simulink model "simulator"  (R2024a)
settings: Solver=VariableStepAuto  StartTime=0.0  StopTime=10  RelTol=1e-3
values from neighbouring files (symbols this model uses):
  params = struct()    [Data.m]
libraries: simulink x2, matrix_library x1
settings Model: Creator=matteocolussi  LastModifiedBy=matteocolussi

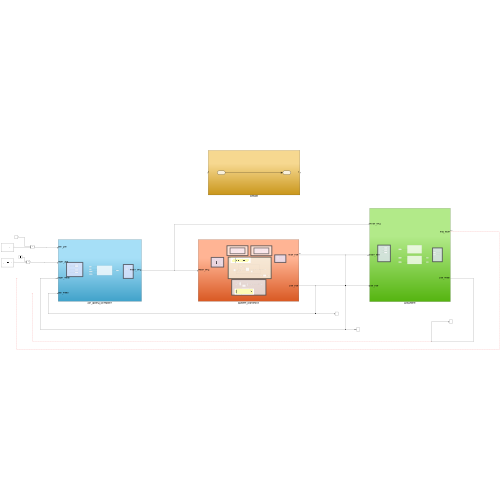
[thumbnail: Simulink's stored preview of the top-level diagram]
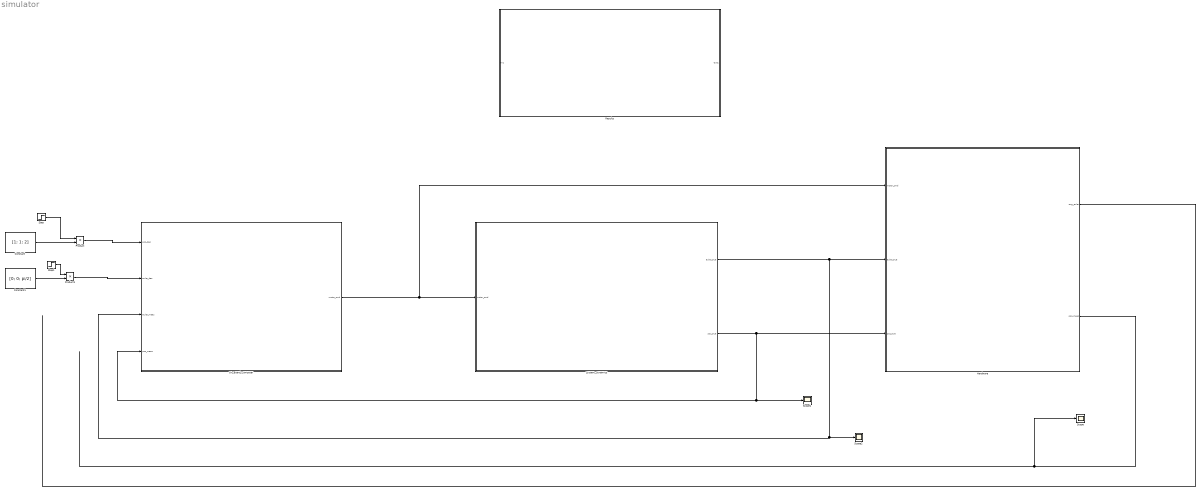
== system simulator ==
  Constant : Constant  Value=[1; 1; 2]
  Constant1 : Constant  Value=[0; 0; pi/2]
  Hardware : Subsystem
  On_Board_Computer : Subsystem
  Product : Product
  Product1 : Product
  Results : Subsystem
  Scope : Scope
  Scope1 : Scope
  Scope2 : Scope
  Step : Step  Time=0  SampleTime=0
  Step1 : Step  Time=0  SampleTime=0
  System_Dynamics : Subsystem
  wires:
  On_Board_Computer/1(motor_cmd) -> Hardware/1(motor_cmd), System_Dynamics/1(motor_cmd)
  System_Dynamics/1(euler_true) -> Hardware/2(euler_true), On_Board_Computer/3(euler_meas), Scope2/1
  System_Dynamics/2(pos_true) -> Scope1/1, On_Board_Computer/4(pos_meas), Hardware/3(pos_true)
  Hardware/1(ang_euler) -> ?
  Hardware/2(pos_meas) -> Scope/1
  Constant/1 -> Product/2
  Step/1 -> Product/1
  Product/1 -> On_Board_Computer/1(pos_des)
  Constant1/1 -> Product1/2
  Step1/1 -> Product1/1
  Product1/1 -> On_Board_Computer/2(euler_des)

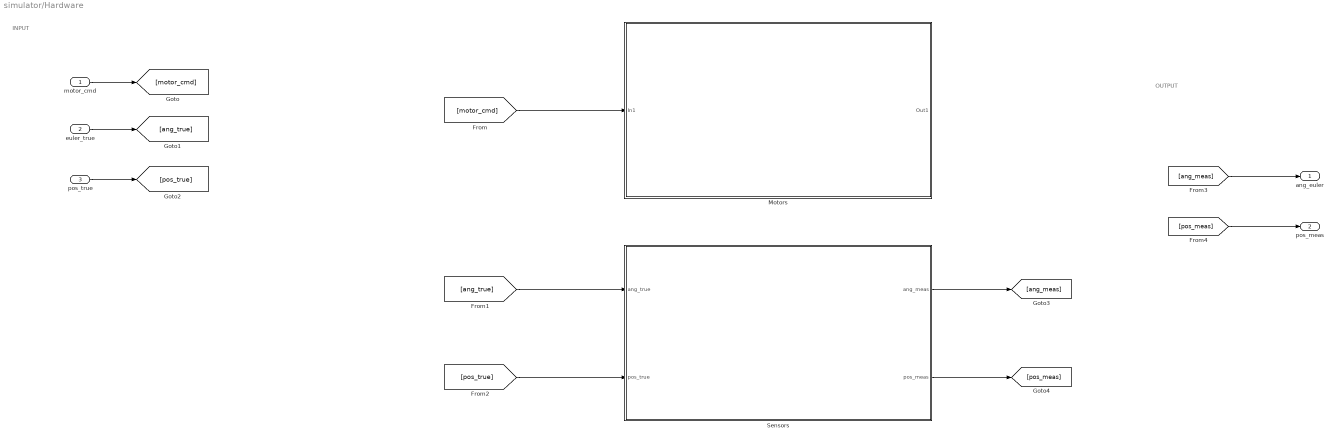
== system simulator/Hardware ==
  note: INPUT
  note: OUTPUT
  motor_cmd : Inport
  euler_true : Inport  Port=2
  pos_true : Inport  Port=3
  Motors : Subsystem
  Sensors : Subsystem
  ang_euler : Outport
  pos_meas : Outport  Port=2
  wires:
  motor_cmd/1 -> [motor_cmd]
  [motor_cmd] -> Motors/1(In1)
  euler_true/1 -> [ang_true]
  pos_true/1 -> [pos_true]
  [ang_true] -> Sensors/1(ang_true)
  [pos_true] -> Sensors/2(pos_true)
  Sensors/1(ang_meas) -> [ang_meas]
  Sensors/2(pos_meas) -> [pos_meas]
  [ang_meas] -> ang_euler/1
  [pos_meas] -> pos_meas/1

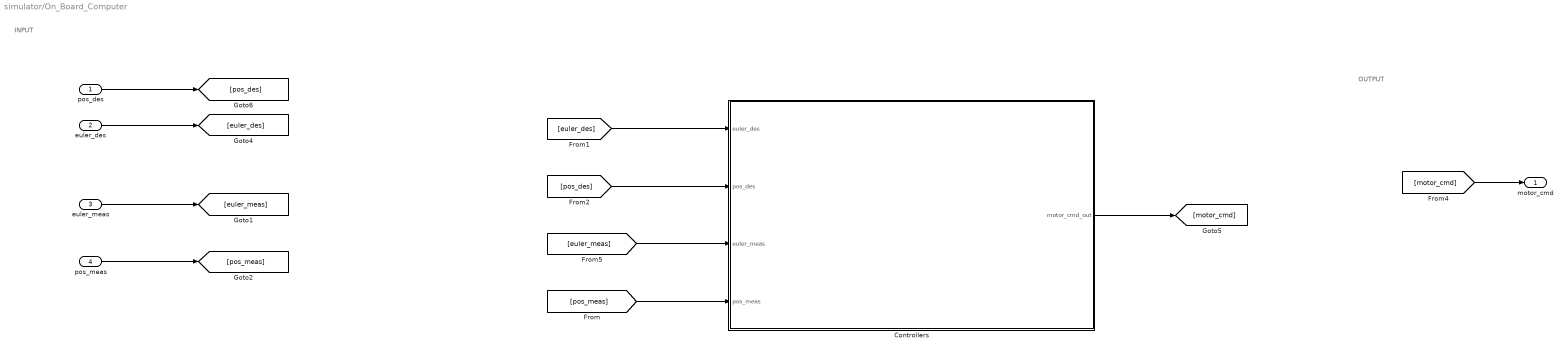
== system simulator/On_Board_Computer ==
  note: OUTPUT
  note: INPUT
  pos_des : Inport
  euler_des : Inport  Port=2
  euler_meas : Inport  Port=3
  pos_meas : Inport  Port=4
  Controllers : Subsystem
  motor_cmd : Outport
  wires:
  pos_des/1 -> [pos_des]
  [euler_des] -> Controllers/1(euler_des)
  [pos_des] -> Controllers/2(pos_des)
  euler_des/1 -> [euler_des]
  Controllers/1(motor_cmd_out) -> [motor_cmd]
  [motor_cmd] -> motor_cmd/1
  euler_meas/1 -> [euler_meas]
  pos_meas/1 -> [pos_meas]
  [pos_meas] -> Controllers/4(pos_meas)
  [euler_meas] -> Controllers/3(euler_meas)

== system simulator/Results ==
  In1 : Inport
  Out1 : Outport
  wires:
  In1/1 -> Out1/1

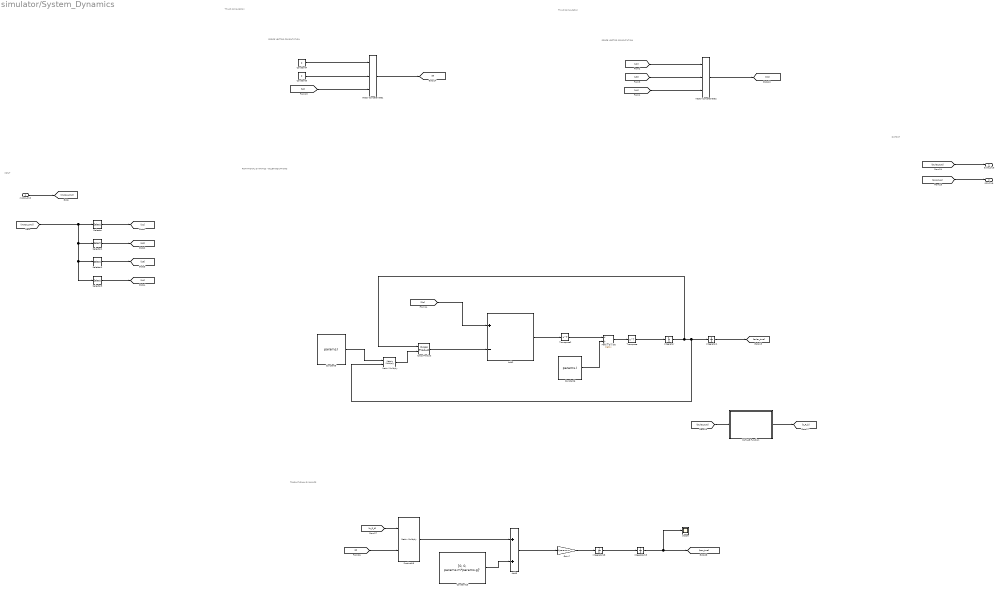
== system simulator/System_Dynamics ==
  note: ROTATIONAL DYNAMICS - EULER EQUATIONS
  note: FORCE VECTOR COMPUTATION
  note: Thrust computation
  note: INPUT
  note: OUTPUT
  note: TRASLATIONAL DYNAMICS
  note: Thrust computation
  note: FORCE VECTOR COMPUTATION
  motor_cmd : Inport
  Add2 : Sum  Inputs=+-
  Add6 : Sum
  Constant13 : Constant  Value=[0, 0, params.m*params.g]'
  Constant3 : Constant  Value=0
  Constant4 : Constant  Value=0
  Constant5 : Constant  Value=params.I  VectorParams1D=off
  Constant6 : Constant  Value=params.I
  Cross Product : matrix_library/Cross Product
  Gain7 : Gain  Gain=1/params.m
  Integrator{,1,18..19} (4 alike) : Integrator
  MATLAB Function : MATLAB Function  TreatAsAtomicUnit=on
  Matrix Divide : Product  Inputs=*/  Multiplication=Matrix(*)
  Matrix Multiply : Product  Multiplication=Matrix(*)
  Product18 : Product  Multiplication=Matrix(*)
  Scope : Scope
  Selector : Selector  InputPortWidth=4  IndexOptions=Index vector (dialog)  Indices=1  OutputSizes=1
  Selector1 : Selector  InputPortWidth=4  IndexOptions=Index vector (dialog)  Indices=2  OutputSizes=1
  Selector2 : Selector  InputPortWidth=4  IndexOptions=Index vector (dialog)  Indices=3  OutputSizes=1
  Selector3 : Selector  InputPortWidth=4  IndexOptions=Index vector (dialog)  Indices=4  OutputSizes=1
  Transpose : Math  Operator=transpose
  Transpose2 : Math  Operator=transpose
  Vector Concatenate1 : Concatenate  NumInputs=3
  Vector Concatenate2 : Concatenate  NumInputs=3
  euler_true : Outport
  pos_true : Outport  Port=2
  wires:
  motor_cmd/1 -> [motor_cmd]
  Selector/1 -> [U1]
  Selector1/1 -> [U2]
  Selector2/1 -> [U3]
  [motor_cmd] -> Selector3/1, Selector2/1, Selector1/1, Selector/1
  Selector3/1 -> [U4]
  [U1] -> Vector Concatenate1/3
  Constant3/1 -> Vector Concatenate1/2
  Constant4/1 -> Vector Concatenate1/1
  Vector Concatenate1/1 -> [F]  "Force"
  [euler_true] -> MATLAB Function/1(ang)
  MATLAB Function/1(o_R_b) -> [o_R_b]
  [euler_true] -> euler_true/1
  [pos_true] -> pos_true/1
  Add6/1 -> Gain7/1
  [F] -> Product18/2
  Product18/1 -> Add6/1
  Gain7/1 -> Integrator18/1  "r_dotdot"
  [o_R_b] -> Product18/1
  Constant13/1 -> Add6/2
  Integrator18/1 -> Integrator19/1  "r_dot"
  Integrator19/1 -> [pos_true], Scope/1  "r"
  Constant5/1 -> Matrix Multiply/1
  Matrix Multiply/1 -> Cross Product/2
  Cross Product/1 -> Add2/2
  Add2/1 -> Transpose2/1
  Constant6/1 -> Matrix Divide/2
  Matrix Divide/1 -> Transpose/1  "w_dot"
  Integrator/1 -> Cross Product/1, Matrix Multiply/2, Integrator1/1  "w"
  Integrator1/1 -> [euler_true]  "euler_angles"
  [U2] -> Vector Concatenate2/1
  Vector Concatenate2/1 -> [Mc]  "Torque"
  [U4] -> Vector Concatenate2/3
  [U3] -> Vector Concatenate2/2
  Transpose/1 -> Integrator/1
  [Mc] -> Add2/1
  Transpose2/1 -> Matrix Divide/1

== system simulator/Hardware/Motors ==
  In1 : Inport
  Out1 : Outport
  wires:
  In1/1 -> Out1/1

== system simulator/Hardware/Sensors ==
  note: OUTPUT
  note: INPUT
  ang_true : Inport
  pos_true : Inport  Port=2
  MPU6050 : Subsystem
  ang_meas : Outport
  pos_meas : Outport  Port=2
  wires:
  ang_true/1 -> [ang_true]
  pos_true/1 -> [pos_true]
  [ang_meas] -> ang_meas/1
  [pos_meas] -> pos_meas/1
  [ang_true] -> MPU6050/1(ang_true)
  [pos_true] -> MPU6050/2(pos_true)
  MPU6050/1(ang_meas) -> [ang_meas]
  MPU6050/2(pos_meas) -> [pos_meas]

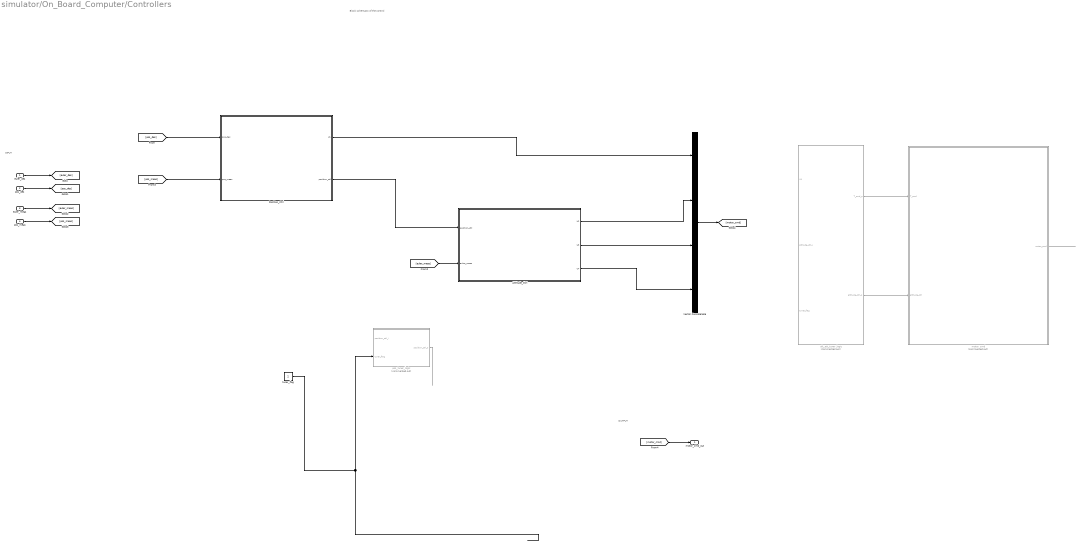
== system simulator/On_Board_Computer/Controllers ==
  note: Block schematic of the control
  note: OUTPUT
  note: INPUT
  euler_des : Inport
  pos_des : Inport  Port=2
  euler_meas : Inport  Port=3
  pos_meas : Inport  Port=4
  Attitude_Ctrl : Subsystem
  Position_Ctrl : Subsystem
  Vector Concatenate : Concatenate  NumInputs=4
  alt_att_tuner_logic : Subsystem  Commented=on
  motor_cmd : Subsystem  Commented=on
  pos_tuner_logic : Subsystem  Commented=on
  tuner_flag : Constant  Value=2
  motor_cmd_out : Outport
  wires:
  euler_des/1 -> [euler_des]
  pos_des/1 -> [pos_des]
  pos_meas/1 -> [pos_meas]
  euler_meas/1 -> [euler_meas]
  [euler_meas] -> Attitude_Ctrl/2(euler_meas)
  motor_cmd/1(motor_cmd) -> ?
  [motor_cmd] -> motor_cmd_out/1
  [pos_meas] -> Position_Ctrl/2(pos_meas)
  tuner_flag/1 -> pos_tuner_logic/2(tuner_flag)
  [pos_des] -> Position_Ctrl/1(pos_des)
  Position_Ctrl/2(position_ctrl) -> Attitude_Ctrl/1(position_ctrl)
  pos_tuner_logic/1(position_ctrl_o) -> ?
  Position_Ctrl/1(U1) -> Vector Concatenate/1
  alt_att_tuner_logic/1(T_cmd_o) -> motor_cmd/1(T_cmd)
  alt_att_tuner_logic/2(attitude_ctrl_o) -> motor_cmd/2(attitude_ctrl)
  Attitude_Ctrl/1(U2) -> Vector Concatenate/2
  Attitude_Ctrl/2(U3) -> Vector Concatenate/3
  Attitude_Ctrl/3(U4) -> Vector Concatenate/4
  Vector Concatenate/1 -> [motor_cmd]

== system simulator/Hardware/Sensors/MPU6050 ==
  note: INPUT
  note: OUTPUT
  ang_true : Inport
  pos_true : Inport  Port=2
  ACCELEROMETER : Subsystem
  GYROSCOPE : Subsystem
  ang_meas : Outport
  pos_meas : Outport  Port=2
  wires:
  ang_true/1 -> [ang_true]
  pos_true/1 -> [pos_true]
  [pos_meas] -> pos_meas/1
  [ang_meas] -> ang_meas/1
  [ang_true] -> GYROSCOPE/1(ang_true)
  [pos_true] -> ACCELEROMETER/1(pos_true)
  GYROSCOPE/1(ang_meas) -> [ang_meas]
  ACCELEROMETER/1(pos_meas) -> [pos_meas]

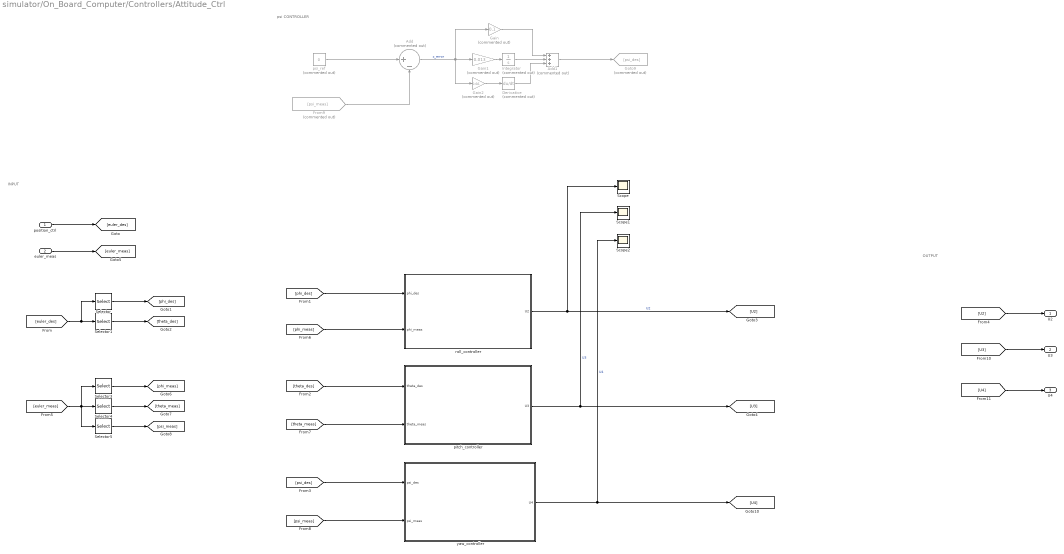
== system simulator/On_Board_Computer/Controllers/Attitude_Ctrl ==
  note: OUTPUT
  note: INPUT
  note: psi CONTROLLER
  position_ctrl : Inport
  euler_meas : Inport  Port=2
  Add : Sum  Commented=on  Inputs=|+-
  Add1 : Sum  Commented=on  Inputs=+++
  Derivative : Derivative  Commented=on
  From9 : From  Commented=on  GotoTag=psi_meas
  Gain : Gain  Commented=on  Gain=0.1
  Gain1 : Gain  Commented=on  Gain=0.013
  Gain2 : Gain  Commented=on  Gain=0.66
  Goto9 : Goto  Commented=on  GotoTag=psi_des
  Integrator : Integrator  Commented=on
  Scope : Scope
  Scope1 : Scope
  Scope2 : Scope
  Selector : Selector  InputPortWidth=2  IndexOptions=Index vector (dialog)  Indices=1  OutputSizes=1
  Selector1 : Selector  InputPortWidth=2  IndexOptions=Index vector (dialog)  Indices=2  OutputSizes=1
  Selector3 : Selector  InputPortWidth=3  IndexOptions=Index vector (dialog)  Indices=1  OutputSizes=1
  Selector4 : Selector  InputPortWidth=3  IndexOptions=Index vector (dialog)  Indices=2  OutputSizes=1
  Selector5 : Selector  InputPortWidth=3  IndexOptions=Index vector (dialog)  Indices=3  OutputSizes=1
  pitch_controller : Subsystem
  psi_ref : Constant  Commented=on  Value=0
  roll_controller : Subsystem
  yaw_controller : Subsystem
  U2 : Outport
  U3 : Outport  Port=2
  U4 : Outport  Port=3
  wires:
  position_ctrl/1 -> [euler_des]
  [phi_des] -> roll_controller/1(phi_des)
  [theta_des] -> pitch_controller/1(theta_des)
  [psi_des] -> yaw_controller/1(psi_des)
  roll_controller/1(U2) -> [U2], Scope/1  "U2"
  pitch_controller/1(U3) -> [U3], Scope1/1  "U3"
  yaw_controller/1(U4) -> [U4], Scope2/1  "U4"
  euler_meas/1 -> [euler_meas]
  [phi_meas] -> roll_controller/2(phi_meas)
  [theta_meas] -> pitch_controller/2(theta_meas)
  [psi_meas] -> yaw_controller/2(psi_meas)
  Selector/1 -> [phi_des]
  [euler_des] -> Selector1/1, Selector/1
  Selector1/1 -> [theta_des]
  [euler_meas] -> Selector5/1, Selector4/1, Selector3/1
  Selector4/1 -> [theta_meas]
  Selector5/1 -> [psi_meas]
  Selector3/1 -> [phi_meas]
  [U2] -> U2/1
  psi_ref/1 -> Add/1
  From9/1 -> Add/2
  [U3] -> U3/1
  [U4] -> U4/1
  Gain1/1 -> Integrator/1
  Integrator/1 -> Add1/2
  Add/1 -> Gain2/1, Gain1/1, Gain/1  "z_error"
  Add1/1 -> Goto9/1
  Gain/1 -> Add1/1
  Derivative/1 -> Add1/3
  Gain2/1 -> Derivative/1

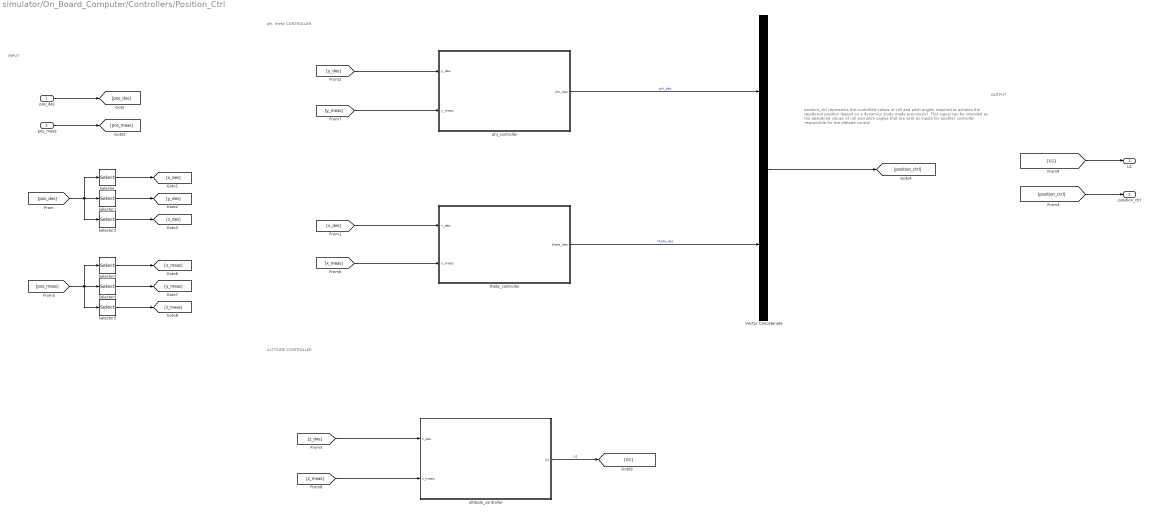
== system simulator/On_Board_Computer/Controllers/Position_Ctrl ==
  note: position_ctrl represents the controlled values of roll and pitch angles required to achieve the desidered position (based on a dynamics study made previously).
      |
      | This signal can be intended as the desidered values of roll and pitch angles that are sent as inputs for another controller, responsible for the attitude control .
  note: ALTITUDE CONTROLLER
  note: phi, theta CONTROLLER
  note: INPUT
  note: OUTPUT
  pos_des : Inport
  pos_meas : Inport  Port=2
  Selector : Selector  InputPortWidth=3  IndexOptions=Index vector (dialog)  Indices=1  OutputSizes=1
  Selector1 : Selector  InputPortWidth=3  IndexOptions=Index vector (dialog)  Indices=2  OutputSizes=1
  Selector2 : Selector  InputPortWidth=3  IndexOptions=Index vector (dialog)  Indices=3  OutputSizes=1
  Selector3 : Selector  InputPortWidth=3  IndexOptions=Index vector (dialog)  Indices=1  OutputSizes=1
  Selector4 : Selector  InputPortWidth=3  IndexOptions=Index vector (dialog)  Indices=2  OutputSizes=1
  Selector5 : Selector  InputPortWidth=3  IndexOptions=Index vector (dialog)  Indices=3  OutputSizes=1
  Vector Concatenate : Concatenate
  altitude_controller : Subsystem
  phi_controller : Subsystem
  theta_controller : Subsystem
  U1 : Outport
  position_ctrl : Outport  Port=2
  wires:
  Selector3/1 -> [x_meas]
  Selector4/1 -> [y_meas]
  [pos_meas] -> Selector5/1, Selector4/1, Selector3/1
  pos_meas/1 -> [pos_meas]
  Selector5/1 -> [z_meas]
  [pos_des] -> Selector2/1, Selector1/1, Selector/1
  Selector/1 -> [x_des]
  pos_des/1 -> [pos_des]
  Selector1/1 -> [y_des]
  Selector2/1 -> [z_des]
  [y_meas] -> phi_controller/2(y_meas)
  [x_des] -> theta_controller/1(x_des)
  [y_des] -> phi_controller/1(y_des)
  [x_meas] -> theta_controller/2(x_meas)
  [position_ctrl] -> position_ctrl/1
  Vector Concatenate/1 -> [position_ctrl]
  theta_controller/1(theta_des) -> Vector Concatenate/2  "theta_des"
  [z_meas] -> altitude_controller/2(z_meas)
  [z_des] -> altitude_controller/1(z_des)
  altitude_controller/1(U1) -> [U1]  "U1"
  [U1] -> U1/1
  phi_controller/1(phi_des) -> Vector Concatenate/1  "phi_des"

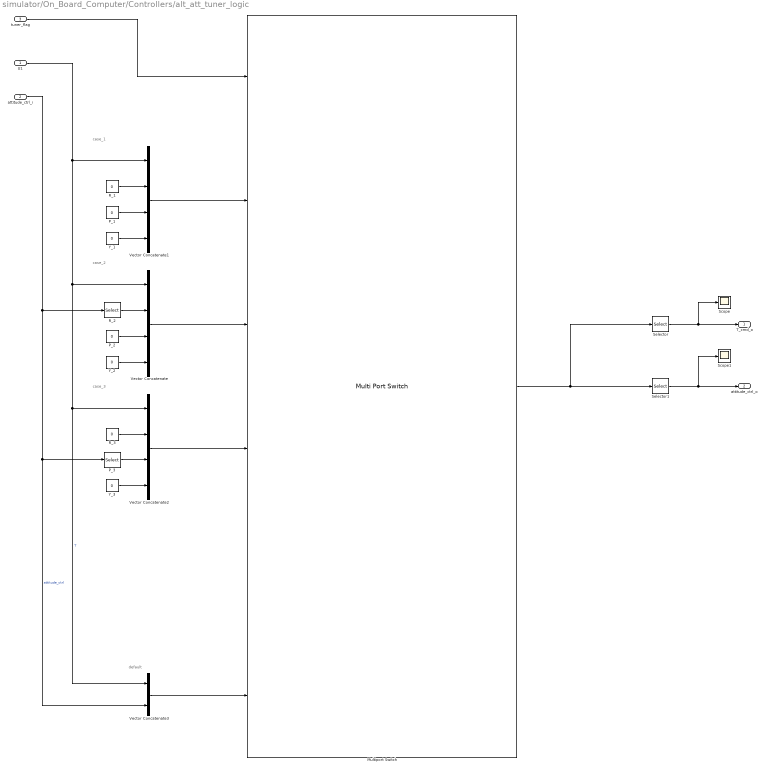
== system simulator/On_Board_Computer/Controllers/alt_att_tuner_logic ==
  note: case_2
  note: case_1
  note: case_3
  note: default
  U1 : Inport
  attitude_ctrl_i : Inport  Port=2
  tuner_flag : Inport  Port=3
  Multiport Switch : MultiPortSwitch  Inputs=5  SaturateOnIntegerOverflow=off  InputSameDT=off
  P_1 : Constant  Value=0
  P_2 : Constant  Value=0
  P_3 : Selector  InputPortWidth=3  IndexOptions=Index vector (dialog)  Indices=2  OutputSizes=1
  R_1 : Constant  Value=0
  R_2 : Selector  InputPortWidth=3  IndexOptions=Index vector (dialog)  Indices=1  OutputSizes=1
  R_3 : Constant  Value=0
  Scope : Scope
  Scope1 : Scope
  Selector : Selector  InputPortWidth=4  IndexOptions=Index vector (dialog)  Indices=1  OutputSizes=1
  Selector1 : Selector  InputPortWidth=4  IndexOptions=Index vector (dialog)  Indices=2:4  OutputSizes=1
  Vector Concatenate : Concatenate  NumInputs=4
  Vector Concatenate1 : Concatenate  NumInputs=4
  Vector Concatenate2 : Concatenate  NumInputs=4
  Vector Concatenate3 : Concatenate
  Y_1 : Constant  Value=0
  Y_2 : Constant  Value=0
  Y_3 : Constant  Value=0
  T_cmd_o : Outport
  attitude_ctrl_o : Outport  Port=2
  wires:
  tuner_flag/1 -> Multiport Switch/1
  Vector Concatenate/1 -> Multiport Switch/3
  P_2/1 -> Vector Concatenate/3
  Y_2/1 -> Vector Concatenate/4
  Multiport Switch/1 -> Selector/1, Selector1/1
  Selector/1 -> Scope/1, T_cmd_o/1
  Selector1/1 -> Scope1/1, attitude_ctrl_o/1
  R_2/1 -> Vector Concatenate/2
  R_1/1 -> Vector Concatenate1/2
  P_1/1 -> Vector Concatenate1/3
  Y_1/1 -> Vector Concatenate1/4
  Vector Concatenate1/1 -> Multiport Switch/2
  P_3/1 -> Vector Concatenate2/3
  Y_3/1 -> Vector Concatenate2/4
  Vector Concatenate2/1 -> Multiport Switch/4
  R_3/1 -> Vector Concatenate2/2
  U1/1 -> Vector Concatenate3/1, Vector Concatenate2/1, Vector Concatenate/1, Vector Concatenate1/1  "T"
  Vector Concatenate3/1 -> Multiport Switch/6
  attitude_ctrl_i/1 -> Vector Concatenate3/2, P_3/1, R_2/1  "attitude_ctrl"

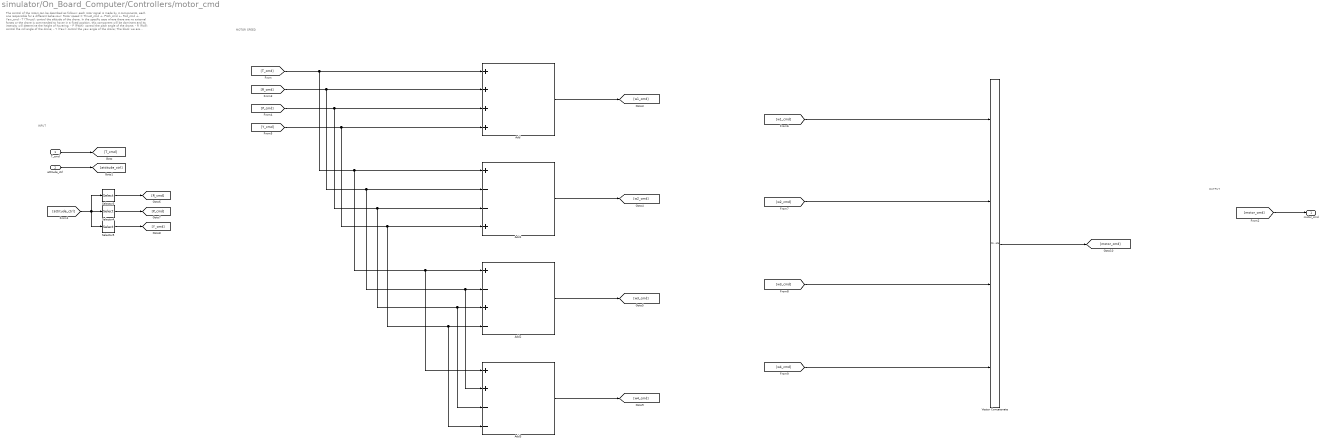
== system simulator/On_Board_Computer/Controllers/motor_cmd ==
  note: The control of the rotors can be described as follows:
      |
      | each rotor signal is made by 4 components, each one responsible for a different behaviour:
      |
      | Rotor speed = Thrust_cmd +- Pitch_cmd +- Roll_cmd +- Yaw_cmd
      |
      | - T (Thrust): control the altitude of the drone. In the specific case where there are no
      | external forces or the drone is commanded to hover in a fixed position,
      | this component will be dominant and its intensity will determine the height
      | of hovering;
      | - P (Pitch): control the pitch angle of the drone;
      | - R (Roll): control the roll angle of the drone;
      | - Y (Yaw): control the yaw angle of the drone;
      |
      | The block we are currently in is responsible for the computation of each component and their correct combination, which is different for every single rotor.
  note: MOTOR SPEED
  note: OUTPUT
  note: INPUT
  T_cmd : Inport
  attitude_ctrl : Inport  Port=2
  Add : Sum  Inputs=++++
  Add1 : Sum  Inputs=+--+
  Add2 : Sum  Inputs=+-+-
  Add3 : Sum  Inputs=++--
  Selector3 : Selector  InputPortWidth=3  IndexOptions=Index vector (dialog)  Indices=1  OutputSizes=1
  Selector4 : Selector  InputPortWidth=3  IndexOptions=Index vector (dialog)  Indices=2  OutputSizes=1
  Selector5 : Selector  InputPortWidth=3  IndexOptions=Index vector (dialog)  Indices=3  OutputSizes=1
  Vector Concatenate : Concatenate  NumInputs=4
  motor_cmd : Outport
  wires:
  T_cmd/1 -> [T_cmd]
  [motor_cmd] -> motor_cmd/1
  attitude_ctrl/1 -> [attitude_ctrl]
  Selector3/1 -> [R_cmd]
  Selector4/1 -> [P_cmd]
  [attitude_ctrl] -> Selector5/1, Selector4/1, Selector3/1
  Selector5/1 -> [Y_cmd]
  [T_cmd] -> Add/1, Add2/1, Add3/1, Add1/1
  [R_cmd] -> Add/2, Add3/2, Add2/2, Add1/2
  [P_cmd] -> Add/3, Add1/3, Add3/3, Add2/3
  [Y_cmd] -> Add/4, Add1/4, Add3/4, Add2/4
  Add/1 -> [w1_cmd]
  Add1/1 -> [w2_cmd]
  Add2/1 -> [w3_cmd]
  Add3/1 -> [w4_cmd]
  Vector Concatenate/1 -> [motor_cmd]
  [w2_cmd] -> Vector Concatenate/2
  [w1_cmd] -> Vector Concatenate/1
  [w3_cmd] -> Vector Concatenate/3
  [w4_cmd] -> Vector Concatenate/4

== system simulator/On_Board_Computer/Controllers/pos_tuner_logic ==
  note: case_2
  note: case_3
  position_ctrl_i : Inport
  tuner_flag : Inport  Port=2
  Multiport Switch : MultiPortSwitch  Inputs=5  SaturateOnIntegerOverflow=off  InputSameDT=off
  Scope : Scope
  Vector Concatenate : Concatenate
  Vector Concatenate1 : Concatenate
  phi_des_2 : Constant  Value=2
  phi_des_3 : Constant  Value=0
  theta_des_2 : Constant  Value=0
  theta_des_3 : Constant  Value=5
  position_ctrl_o : Outport
  wires:
  tuner_flag/1 -> Multiport Switch/1
  Multiport Switch/1 -> Scope/1, position_ctrl_o/1
  position_ctrl_i/1 -> Multiport Switch/6
  Vector Concatenate/1 -> Multiport Switch/3
  phi_des_2/1 -> Vector Concatenate/1
  theta_des_2/1 -> Vector Concatenate/2
  theta_des_3/1 -> Vector Concatenate1/2
  phi_des_3/1 -> Vector Concatenate1/1
  Vector Concatenate1/1 -> Multiport Switch/4

== system simulator/Hardware/Sensors/MPU6050/ACCELEROMETER ==
  pos_true : Inport
  Band-Limited White Noise : simulink/Sources/Band-Limited White Noise  Cov=[0.1]  Ts=0.1  seed=[23341]
  Sum : Sum  Inputs=|++
  pos_meas : Outport
  wires:
  Band-Limited White Noise/1 -> Sum/2
  pos_true/1 -> Sum/1
  Sum/1 -> pos_meas/1

== system simulator/Hardware/Sensors/MPU6050/GYROSCOPE ==
  ang_true : Inport
  Band-Limited White Noise : simulink/Sources/Band-Limited White Noise  Cov=[0.1]  Ts=0.1  seed=[23341]
  Sum : Sum  Inputs=|++
  ang_meas : Outport
  wires:
  ang_true/1 -> Sum/1
  Band-Limited White Noise/1 -> Sum/2
  Sum/1 -> ang_meas/1

== system simulator/On_Board_Computer/Controllers/Attitude_Ctrl/pitch_controller ==
  note: OUTPUT
  note: INPUT
  theta_des : Inport
  theta_meas : Inport  Port=2
  Add : Sum  Inputs=|+-
  Add1 : Sum  Inputs=+++
  Derivative : Derivative
  Gain : Gain
  Gain1 : Gain  Gain=0.13
  Gain2 : Gain  Gain=0.66
  Integrator : Integrator
  U3 : Outport
  wires:
  [U3] -> U3/1
  [theta_des] -> Add/1
  theta_des/1 -> [theta_des]
  theta_meas/1 -> [theta_meas]
  [theta_meas] -> Add/2
  Integrator/1 -> Add1/2
  Gain1/1 -> Integrator/1
  Add/1 -> Gain2/1, Gain1/1, Gain/1  "z_error"
  Gain/1 -> Add1/1
  Derivative/1 -> Add1/3
  Add1/1 -> [U3]
  Gain2/1 -> Derivative/1

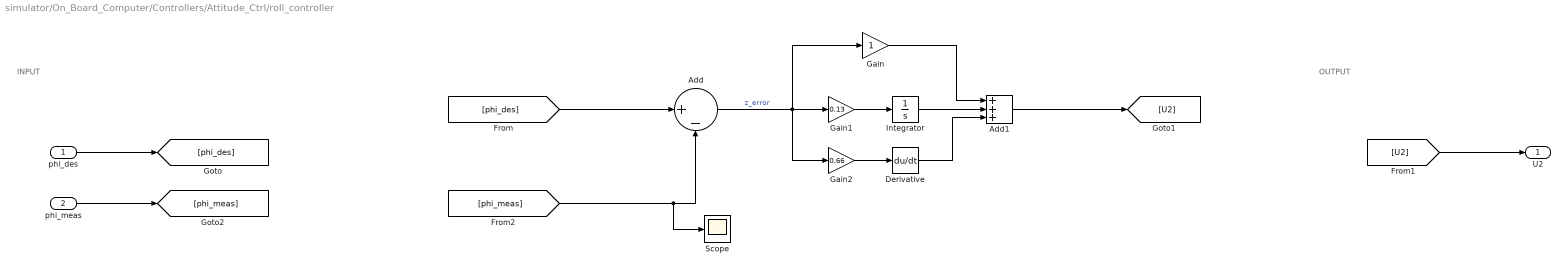
== system simulator/On_Board_Computer/Controllers/Attitude_Ctrl/roll_controller ==
  note: OUTPUT
  note: INPUT
  phi_des : Inport
  phi_meas : Inport  Port=2
  Add : Sum  Inputs=|+-
  Add1 : Sum  Inputs=+++
  Derivative : Derivative
  Gain : Gain
  Gain1 : Gain  Gain=0.13
  Gain2 : Gain  Gain=0.66
  Integrator : Integrator
  Scope : Scope
  U2 : Outport
  wires:
  phi_des/1 -> [phi_des]
  [U2] -> U2/1
  phi_meas/1 -> [phi_meas]
  [phi_meas] -> Scope/1, Add/2
  Integrator/1 -> Add1/2
  Gain1/1 -> Integrator/1
  Add/1 -> Gain2/1, Gain1/1, Gain/1  "z_error"
  Gain/1 -> Add1/1
  Derivative/1 -> Add1/3
  Add1/1 -> [U2]
  Gain2/1 -> Derivative/1
  [phi_des] -> Add/1

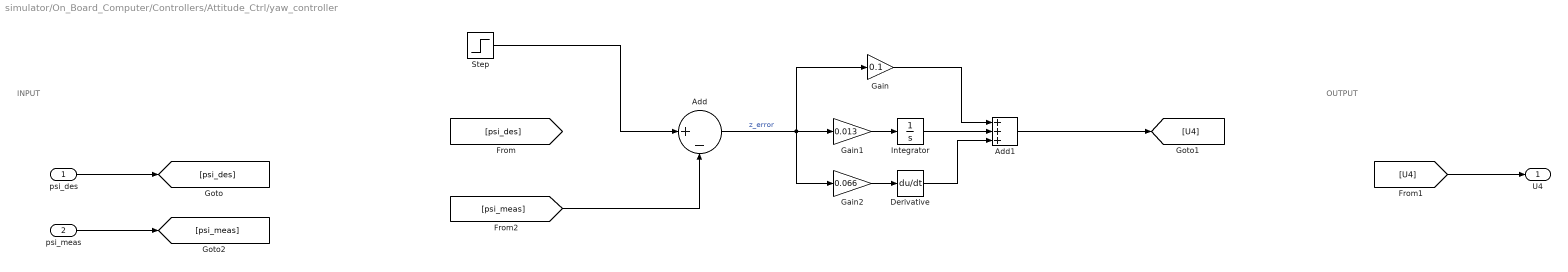
== system simulator/On_Board_Computer/Controllers/Attitude_Ctrl/yaw_controller ==
  note: OUTPUT
  note: INPUT
  psi_des : Inport
  psi_meas : Inport  Port=2
  Add : Sum  Inputs=|+-
  Add1 : Sum  Inputs=+++
  Derivative : Derivative
  Gain : Gain  Gain=0.1
  Gain1 : Gain  Gain=0.013
  Gain2 : Gain  Gain=0.066
  Integrator : Integrator
  Step : Step  Time=0  After=pi/2  SampleTime=0
  U4 : Outport
  wires:
  [U4] -> U4/1
  psi_des/1 -> [psi_des]
  psi_meas/1 -> [psi_meas]
  [psi_meas] -> Add/2
  Integrator/1 -> Add1/2
  Gain1/1 -> Integrator/1
  Add/1 -> Gain2/1, Gain1/1, Gain/1  "z_error"
  Gain/1 -> Add1/1
  Derivative/1 -> Add1/3
  Add1/1 -> [U4]
  Gain2/1 -> Derivative/1
  Step/1 -> Add/1

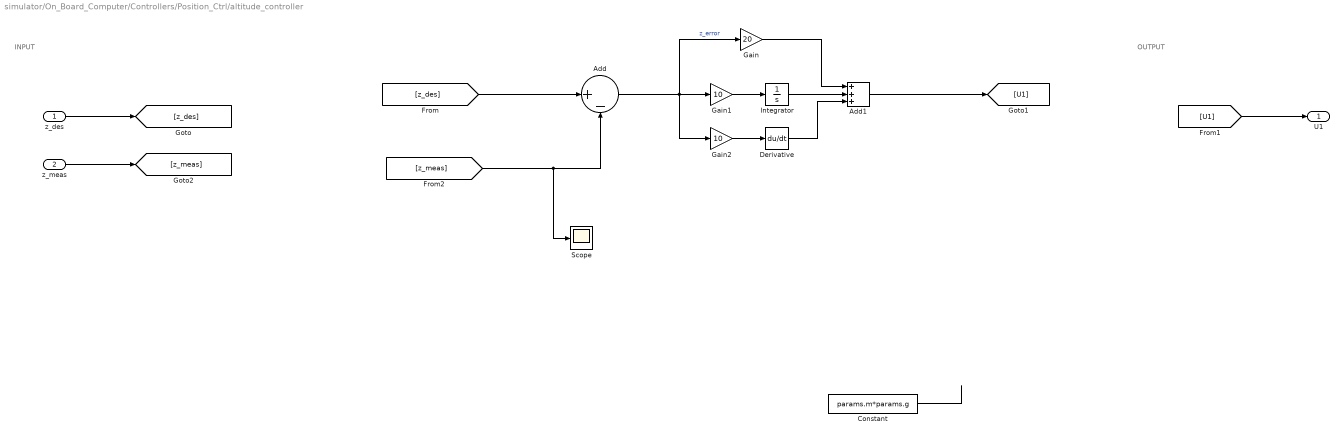
== system simulator/On_Board_Computer/Controllers/Position_Ctrl/altitude_controller ==
  note: OUTPUT
  note: INPUT
  z_des : Inport
  z_meas : Inport  Port=2
  Add : Sum  Inputs=|+-
  Add1 : Sum  Inputs=+++
  Constant : Constant  Value=params.m*params.g
  Derivative : Derivative
  Gain : Gain  Gain=20
  Gain1 : Gain  Gain=10
  Gain2 : Gain  Gain=10
  Integrator : Integrator
  Scope : Scope
  U1 : Outport
  wires:
  [U1] -> U1/1
  z_des/1 -> [z_des]
  z_meas/1 -> [z_meas]
  Add/1 -> Gain2/1, Gain1/1, Gain/1  "z_error"
  [z_meas] -> Scope/1, Add/2
  Add1/1 -> [U1]
  Constant/1 -> ?
  Gain1/1 -> Integrator/1
  Gain/1 -> Add1/1
  Integrator/1 -> Add1/2
  Gain2/1 -> Derivative/1
  Derivative/1 -> Add1/3
  [z_des] -> Add/1

== system simulator/On_Board_Computer/Controllers/Position_Ctrl/phi_controller ==
  note: OUTPUT
  note: INPUT
  y_des : Inport
  y_meas : Inport  Port=2
  Add : Sum  Inputs=|+-
  Add1 : Sum  Inputs=+++
  Derivative : Derivative
  Gain : Gain  Gain=0
  Gain1 : Gain  Gain=0
  Gain2 : Gain  Gain=0
  Integrator : Integrator
  phi_des : Outport
  wires:
  [phi_des] -> phi_des/1
  [y_des] -> Add/1
  y_des/1 -> [y_des]
  y_meas/1 -> [y_meas]
  [y_meas] -> Add/2
  Integrator/1 -> Add1/2
  Gain1/1 -> Integrator/1
  Add/1 -> Gain2/1, Gain1/1, Gain/1
  Gain/1 -> Add1/1
  Derivative/1 -> Add1/3
  Add1/1 -> [phi_des]
  Gain2/1 -> Derivative/1

== system simulator/On_Board_Computer/Controllers/Position_Ctrl/theta_controller ==
  note: OUTPUT
  note: INPUT
  x_des : Inport
  x_meas : Inport  Port=2
  Add : Sum  Inputs=|+-
  Add1 : Sum  Inputs=+++
  Derivative : Derivative
  Gain : Gain  Gain=0
  Gain1 : Gain  Gain=0
  Gain2 : Gain  Gain=0
  Integrator : Integrator
  theta_des : Outport
  wires:
  x_des/1 -> [x_des]
  [x_des] -> Add/1
  [theta_des] -> theta_des/1
  x_meas/1 -> [x_meas]
  [x_meas] -> Add/2
  Integrator/1 -> Add1/2
  Gain1/1 -> Integrator/1
  Add/1 -> Gain2/1, Gain1/1, Gain/1  "z_error"
  Gain/1 -> Add1/1
  Derivative/1 -> Add1/3
  Add1/1 -> [theta_des]
  Gain2/1 -> Derivative/1

== matlab function simulator/System_Dynamics/MATLAB Function ==
  data: ang input; o_R_b output
function o_R_b  = RotMatrix(ang)

phi = ang(1);
theta = ang(2);
psi = ang(3);

o_R_b = zeros(3,3);

R_psi = [cos(psi),          -sin(psi),          0;
         sin(psi),           cos(psi),          0;
                0,                  0,          1];

R_theta = [cos(theta),              0,          sin(theta);
                    0,              1,                   0;
          -sin(theta),              0,          cos(theta)];

R_phi = [1,             0,              0;
         0,      cos(phi),      -sin(phi);
         0,      sin(phi),       cos(phi)];

o_R_b = R_psi * R_theta * R_phi;

end
